simulink model "Blocks"  (R2019a)
settings: Solver=VariableStepAuto  StartTime=0.0  StopTime=10.0  RelTol=1e-3
values from neighbouring files (symbols this model uses):
  A = [0 1;g/l 0]    [PIDtest.m]    (also in SelfBalanceScript.m = [0      1              0           0)
  B = [0;1]    [PIDtest.m]    (also in SelfBalanceScript.m = [0; (I+m*l^2)/p; 0; m*l/p])
  C = [1 0]    [PIDtest.m]    (also in PendulumTF.m = pid(Kp,Ki,Kd); SelfBalanceScript.m = [1 0 0 0)
  K = [k1;k2]    [PIDtest.m]    (also in SelfBalanceScript.m = lqr(A,B,Q,R))
  x0 = [0; 0; 100; 0]    [SelfBalanceScript.m]
settings Model: Creator=jornellq  LastModifiedBy=jornellq

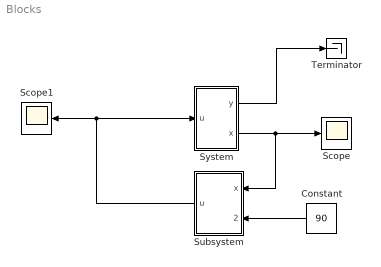
== system Blocks ==
  Constant : Constant  Value=90
  Scope : Scope
  Scope1 : Scope
  Subsystem : Subsystem
  "System " : Subsystem
  Terminator : Terminator
  wires:
  "System "/1(y) -> Terminator/1
  "System "/2(x) -> Subsystem/1(x), Scope/1
  Subsystem/1(u) -> Scope1/1, "System "/1(u)
  Constant/1 -> Subsystem/2(des_pos)

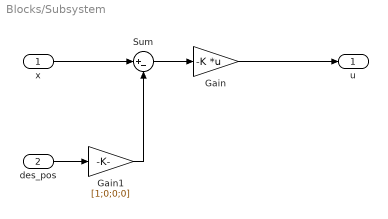
== system Blocks/Subsystem ==
  x : Inport
  des_pos : Inport  Port=2
  Gain : Gain  Gain=-K  Multiplication=Matrix(K*u)
  Gain1 : Gain  Gain=[1;0;0;0]
  Sum : Sum  Inputs=|+-
  u : Outport
  wires:
  Gain/1 -> u/1
  x/1 -> Sum/1
  Sum/1 -> Gain/1
  des_pos/1 -> Gain1/1
  Gain1/1 -> Sum/2

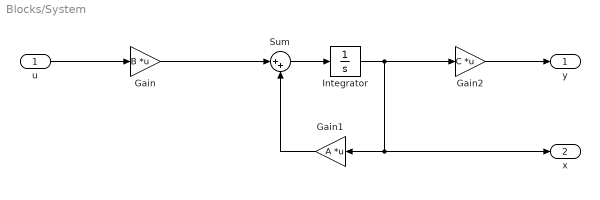
== system Blocks/System  ==
  u : Inport
  Gain : Gain  Gain=B  Multiplication=Matrix(K*u)
  Gain1 : Gain  Gain=A  Multiplication=Matrix(K*u)
  Gain2 : Gain  Gain=C  Multiplication=Matrix(K*u)
  Integrator : Integrator  InitialCondition=x0
  Sum : Sum  Inputs=|++
  y : Outport
  x : Outport  Port=2
  wires:
  u/1 -> Gain/1
  Gain2/1 -> y/1
  Gain/1 -> Sum/1
  Sum/1 -> Integrator/1
  Gain1/1 -> Sum/2
  Integrator/1 -> Gain2/1, Gain1/1, x/1
